simulink model "OperationalSpaceInverseDynamic"  (R2020b)
settings: Solver=VariableStepAuto  StartTime=0.0  StopTime=5  RelTol=1e-3
values from neighbouring files (symbols this model uses):
  KD = diag([  49   100   160    19     0   60])    [parameters.m]
  KP = diag([ 900  3000  1600  100  1  300])    [parameters.m]
libraries: vrlib x1
settings Model: Creator=Edoardo  LastModifiedBy=Edoardo

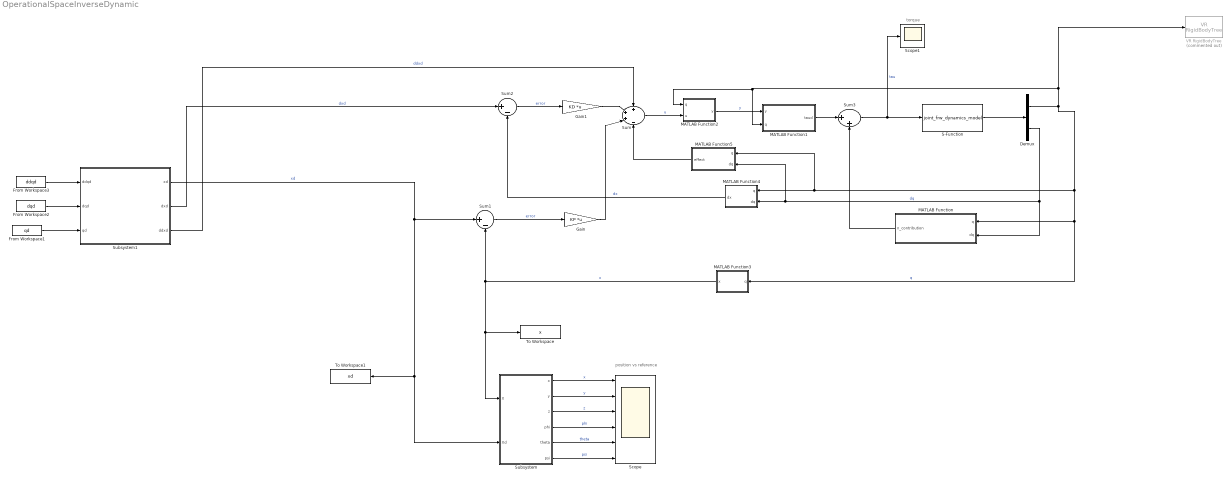
== system OperationalSpaceInverseDynamic ==
  note: torque
  note: position vs reference
  Demux : Demux  Outputs=2
  From Workspace1 : FromWorkspace  VariableName=qd
  From Workspace2 : FromWorkspace  VariableName=dqd
  From Workspace3 : FromWorkspace  VariableName=ddqd
  Gain : Gain  Gain=KP  Multiplication=Matrix(K*u) (u vector)
  Gain1 : Gain  Gain=KD  Multiplication=Matrix(K*u) (u vector)
  MATLAB Function : MATLAB Function  TreatAsAtomicUnit=on
  MATLAB Function1 : MATLAB Function  TreatAsAtomicUnit=on
  MATLAB Function2 : MATLAB Function  TreatAsAtomicUnit=on
  MATLAB Function3 : MATLAB Function  TreatAsAtomicUnit=on
  MATLAB Function4 : MATLAB Function  TreatAsAtomicUnit=on
  MATLAB Function5 : MATLAB Function  TreatAsAtomicUnit=on
  S-Function : S-Function  FunctionName=joint_frw_dynamics_model  Parameters=myRobot  SFunctionDeploymentMode=off  EnableBusSupport=off
  Scope : Scope  NumInputPorts=6
  Scope1 : Scope
  Subsystem : Subsystem
  Subsystem1 : Subsystem
  Sum : Sum  Inputs=+++-
  Sum1 : Sum  Inputs=|+-
  Sum2 : Sum  Inputs=|+-
  Sum3 : Sum  Inputs=|++
  To Workspace : ToWorkspace  VariableName=x  SaveFormat=Timeseries  SampleTime=-1
  To Workspace1 : ToWorkspace  VariableName=xd  SaveFormat=Timeseries  SampleTime=-1
  VR RigidBodyTree : vrlib/VR RigidBodyTree  Commented=on  RBT=robot  useRBT=on  Ts=-1  ForceViewerOpen=on
      settings: SourceProductBaseCode=SL
  wires:
  Gain1/1 -> Sum/2
  Gain/1 -> Sum/3
  Sum2/1 -> Gain1/1  "error"
  Sum1/1 -> Gain/1  "error"
  S-Function/1 -> Demux/1
  Sum3/1 -> S-Function/1, Scope1/1  "tau"
  MATLAB Function/1(n_contribution) -> Sum3/2
  MATLAB Function1/1(taud) -> Sum3/1
  Demux/2 -> MATLAB Function/2(dq), MATLAB Function4/2(dq), MATLAB Function5/2(dq)  "dq"
  Subsystem1/2(dxd) -> Sum2/1  "dxd"
  Demux/1 -> MATLAB Function4/1(q), MATLAB Function5/1(q), MATLAB Function3/1(q), MATLAB Function/1(q), VR RigidBodyTree/1, MATLAB Function2/1(q), MATLAB Function1/2(q)  "q"
  MATLAB Function2/1(y) -> MATLAB Function1/1(y)  "y"
  MATLAB Function4/1(dx) -> Sum2/2  "dx"
  MATLAB Function5/1(effect) -> Sum/4
  Sum/1 -> MATLAB Function2/2(u)  "u"
  Subsystem/1(x) -> Scope/1  "x"
  Subsystem/4(phi) -> Scope/4  "phi"
  Subsystem/6(psi) -> Scope/6  "psi"
  Subsystem/2(y) -> Scope/2  "y"
  Subsystem/5(theta) -> Scope/5  "theta"
  MATLAB Function3/1(x) -> To Workspace/1, Subsystem/1(X), Sum1/2  "x"
  Subsystem1/1(xd) -> Sum1/1, To Workspace1/1, Subsystem/2(Xd)  "xd"
  Subsystem/3(z) -> Scope/3  "z"
  Subsystem1/3(ddxd) -> Sum/1  "ddxd"
  From Workspace1/1 -> Subsystem1/3(qd)
  From Workspace3/1 -> Subsystem1/1(ddqd)
  From Workspace2/1 -> Subsystem1/2(dqd)

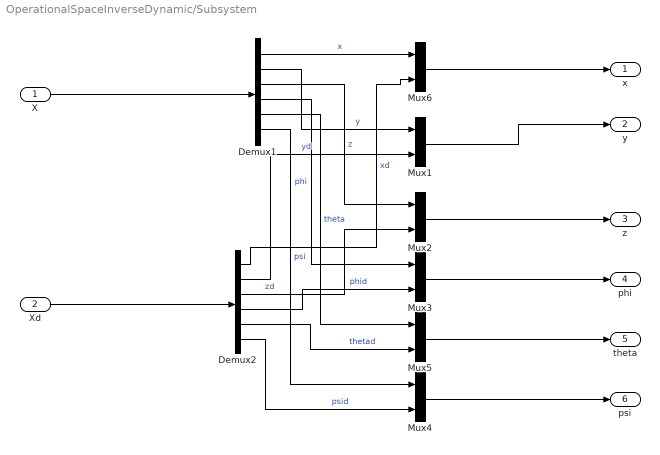
== system OperationalSpaceInverseDynamic/Subsystem ==
  X : Inport
  Xd : Inport  Port=2
  Demux1 : Demux  Outputs=6
  Demux2 : Demux  Outputs=6
  Mux{1..6} (6 alike) : Mux  Inputs=2
  x : Outport
  y : Outport  Port=2
  z : Outport  Port=3
  phi : Outport  Port=4
  theta : Outport  Port=5
  psi : Outport  Port=6
  wires:
  Demux1/3 -> Mux2/1  "z"
  Demux1/4 -> Mux3/1  "phi"
  Demux2/3 -> Mux2/2  "zd"
  Mux2/1 -> z/1
  Demux2/1 -> Mux6/2  "xd"
  Demux1/5 -> Mux5/1  "theta"
  Mux1/1 -> y/1
  Demux1/6 -> Mux4/1  "psi"
  Demux1/1 -> Mux6/1  "x"
  Demux2/5 -> Mux5/2  "thetad"
  Demux2/6 -> Mux4/2  "psid"
  Demux1/2 -> Mux1/1  "y"
  Demux2/4 -> Mux3/2  "phid"
  Demux2/2 -> Mux1/2  "yd"
  Xd/1 -> Demux2/1
  X/1 -> Demux1/1
  Mux3/1 -> phi/1
  Mux5/1 -> theta/1
  Mux4/1 -> psi/1
  Mux6/1 -> x/1

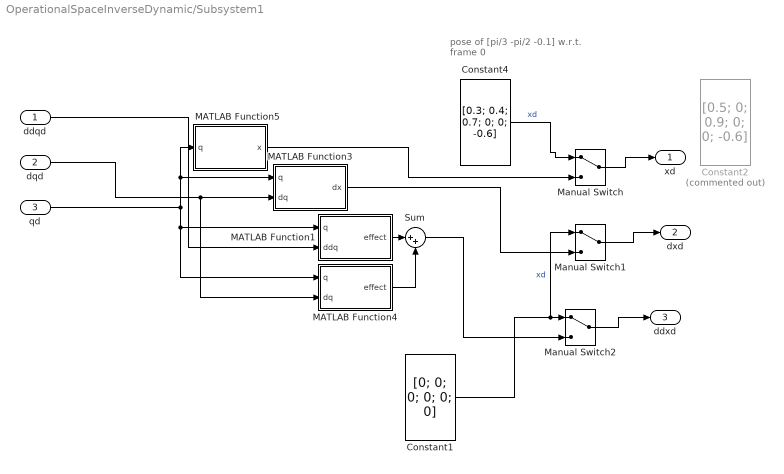
== system OperationalSpaceInverseDynamic/Subsystem1 ==
  note: pose of [pi/3 -pi/2 -0.1]
      | w.r.t. frame 0
  ddqd : Inport
  dqd : Inport  Port=2
  qd : Inport  Port=3
  Constant1 : Constant  Value=[0; 0; 0; 0; 0; 0]  VectorParams1D=off
  Constant2 : Constant  Commented=on  Value=[0.5; 0; 0.9; 0; 0; -0.6]  VectorParams1D=off
  Constant4 : Constant  Value=[0.3; 0.4; 0.7; 0; 0; -0.6]  VectorParams1D=off
  MATLAB Function1 : MATLAB Function  TreatAsAtomicUnit=on
  MATLAB Function3 : MATLAB Function  TreatAsAtomicUnit=on
  MATLAB Function4 : MATLAB Function  TreatAsAtomicUnit=on
  MATLAB Function5 : MATLAB Function  TreatAsAtomicUnit=on
  Manual Switch : ManualSwitch
  Manual Switch1 : ManualSwitch
  Manual Switch2 : ManualSwitch
  Sum : Sum  Inputs=|++
  xd : Outport
  dxd : Outport  Port=2
  ddxd : Outport  Port=3
  wires:
  Sum/1 -> Manual Switch2/2
  qd/1 -> MATLAB Function5/1(q), MATLAB Function3/1(q), MATLAB Function4/1(q), MATLAB Function1/1(q)
  MATLAB Function4/1(effect) -> Sum/2
  MATLAB Function3/1(dx) -> Manual Switch1/2
  dqd/1 -> MATLAB Function3/2(dq), MATLAB Function4/2(dq)
  MATLAB Function1/1(effect) -> Sum/1
  ddqd/1 -> MATLAB Function1/2(ddq)
  MATLAB Function5/1(x) -> Manual Switch/2
  Constant4/1 -> Manual Switch/1  "xd"
  Manual Switch/1 -> xd/1
  Manual Switch1/1 -> dxd/1
  Manual Switch2/1 -> ddxd/1
  Constant1/1 -> Manual Switch1/1, Manual Switch2/1  "xd"

== matlab function OperationalSpaceInverseDynamic/MATLAB Function ==
  data: q input size=3; n_contribution output; dq input size=3
function n_contribution = n(q,dq)
    n_contribution = getCHatLagrangian(q,dq)*dq + getGHatLagrangian(q);

== matlab function OperationalSpaceInverseDynamic/MATLAB Function2 ==
  data: q input; u input; y output
function y = JA_inv(q,u)

y = pinv(getAnalyticalJacobian(q))*u;

== matlab function OperationalSpaceInverseDynamic/MATLAB Function3 ==
  data: q input size=3; x output size=6
function x = K(q)

K = getDirectKinematics(q);

pos = K(1:3, 4);
rotm = K(1:3,1:3); 
ori = rotm2eul(rotm, 'ZYZ')';

x = [pos; ori];

== matlab function OperationalSpaceInverseDynamic/MATLAB Function4 ==
  data: q input size=3; dx output size=6; dq input size=3
function dx = JA(q,dq)

dx = getAnalyticalJacobian(q)*dq;

== matlab function OperationalSpaceInverseDynamic/MATLAB Function5 ==
  data: q input; effect output; dq input
function effect = dJA(q, dq)

    

effect = getDAnalyticalJacobian(q, dq)*dq;

== matlab function OperationalSpaceInverseDynamic/Subsystem1/MATLAB Function3 ==
  data: q input; dx output; dq input
function dx = JA(q, dq)

dx = getAnalyticalJacobian(q)*dq;

== matlab function OperationalSpaceInverseDynamic/Subsystem1/MATLAB Function4 ==
  data: q input; effect output; dq input
function effect = dJA(q, dq)


effect = getDAnalyticalJacobian(q, dq)*dq;

== matlab function OperationalSpaceInverseDynamic/Subsystem1/MATLAB Function5 ==
  data: q input; x output
function x = K(q)

t1 = q(1);
t2 = q(2);
d3 = q(3);

K = [[ cos(t1 + t2), -sin(t1 + t2), 0, (3*cos(t1 + t2))/10 + (2*cos(t1))/5]
     [ sin(t1 + t2),  cos(t1 + t2), 0, (3*sin(t1 + t2))/10 + (2*sin(t1))/5]
     [            0,             0, 1,                            d3 + 2/5]
     [            0,             0, 0,                                   1]];

pos = K(1:3, 4);
ori = rotm2eul(K(1:3,1:3), 'ZYZ')';

x = [pos; ori];

== matlab function OperationalSpaceInverseDynamic/Subsystem1/MATLAB Function1 ==
  data: q input; effect output; ddq input
function effect = JA(q, ddq)

effect = getAnalyticalJacobian(q)*ddq;

== matlab function OperationalSpaceInverseDynamic/MATLAB Function1 ==
  data: y input; taud output; q input size=3
function taud = B(y, q)

    taud = getBHatLagrangian(q)*y;
